simulink model "Test_model"  (R2021a)
settings: Solver=FixedStepDiscrete  StartTime=0.0  StopTime=10  RelTol=1e-3
values from neighbouring files (symbols this model uses):
  ADMM_vec = [ADMM_vec;ADMM_struct]    [Setup.m]
  constraints_struct = [constraints_struct;constraints]    [Setup.m]
undefined symbols (not defined in the file or in its folder): model, Objective
settings Model: SimulationMode=rapid-accelerator  Creator=worc4873  LastModifiedBy=worc4873
settings DebuggingCC: ReadBeforeWriteMsg=DisableAll  WriteAfterWriteMsg=DisableAll  WriteAfterReadMsg=DisableAll  MultiTaskDSMMsg=none
settings ModelReferenceCC: UpdateModelReferenceTargets=IfOutOfDate
settings SFSimCC: SFSimEcho=off

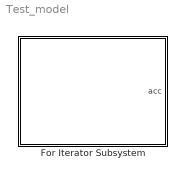
== system Test_model ==
  For Iterator Subsystem : Subsystem  TreatAsAtomicUnit=on

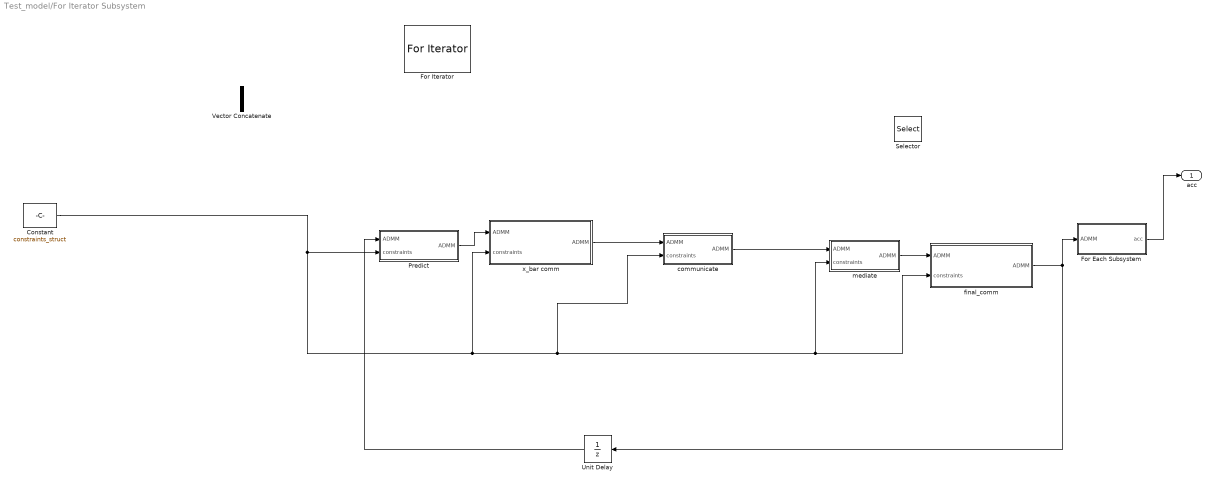
== system Test_model/For Iterator Subsystem ==
  Constant : Constant  Value=constraints_struct  OutDataTypeStr=Bus: constraints
  For Each Subsystem : Subsystem  TreatAsAtomicUnit=on
  For Iterator : ForIterator  IterationLimit=10
  Predict : Subsystem  TreatAsAtomicUnit=on
  Selector : Selector  InputPortWidth=3  IndexOptions=Index vector (dialog)  Indices=[1 3]  OutputSizes=1
  Unit Delay : UnitDelay  InitialCondition=ADMM_vec  SampleTime=-1  HasFrameUpgradeWarning=on
  Vector Concatenate : Concatenate
  communicate : Subsystem  TreatAsAtomicUnit=on
  final_comm : MATLAB Function  TreatAsAtomicUnit=on
  mediate : Subsystem  TreatAsAtomicUnit=on
  x_bar comm : MATLAB Function  TreatAsAtomicUnit=on
  acc : Outport
  wires:
  Constant/1 -> x_bar comm/2(constraints), final_comm/2(constraints), mediate/2(constraints), communicate/2(constraints), Predict/2(constraints)
  Predict/1(ADMM) -> x_bar comm/1("ADMM ")
  Unit Delay/1 -> Predict/1("ADMM ")
  x_bar comm/1(ADMM) -> communicate/1("ADMM ")
  communicate/1(ADMM) -> mediate/1("ADMM ")
  mediate/1(ADMM) -> final_comm/1("ADMM ")
  final_comm/1(ADMM) -> Unit Delay/1, For Each Subsystem/1(ADMM)
  For Each Subsystem/1(acc) -> acc/1

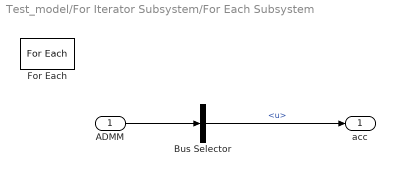
== system Test_model/For Iterator Subsystem/For Each Subsystem ==
  ADMM : Inport  Partition=on  PartitionDimension=1  PartitionWidth=1  PartitionOffset=0
  Bus Selector : BusSelector  OutputSignals=u
  For Each : ForEach  DisableCoverage=on
  acc : Outport  ConcatenationDimension=2
  wires:
  ADMM/1 -> Bus Selector/1
  Bus Selector/1 -> acc/1  "<u>"

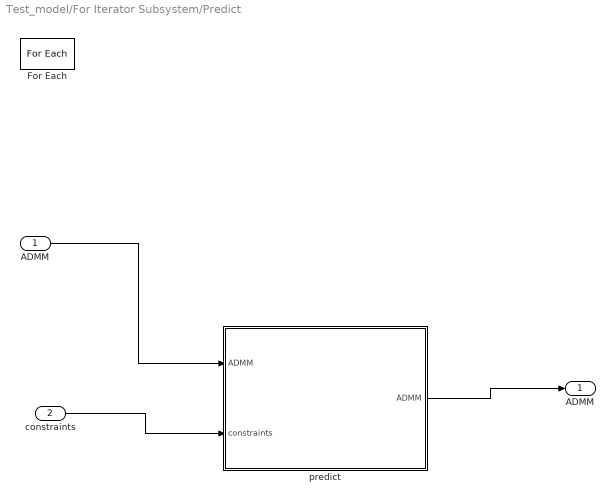
== system Test_model/For Iterator Subsystem/Predict ==
  "ADMM " : Inport  OutDataTypeStr=Bus: ADMM  Partition=on  PartitionDimension=1  PartitionWidth=1  PartitionOffset=0
  constraints : Inport  Port=2  OutDataTypeStr=Bus: constraints  Partition=on  PartitionDimension=1  PartitionWidth=1  PartitionOffset=0
  For Each : ForEach  DisableCoverage=on
  predict : MATLAB Function  TreatAsAtomicUnit=on
  ADMM : Outport  ConcatenationDimension=1
  wires:
  constraints/1 -> predict/2(constraints)
  "ADMM "/1 -> predict/1("ADMM ")
  predict/1(ADMM) -> ADMM/1

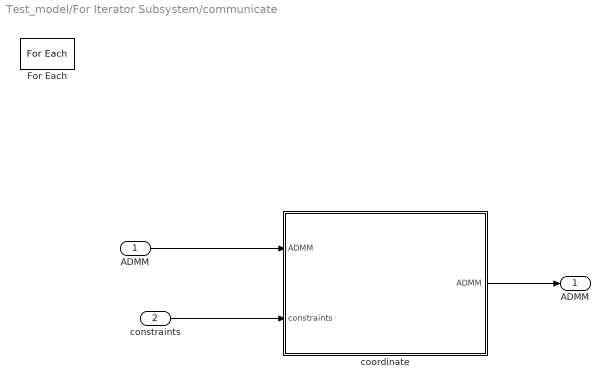
== system Test_model/For Iterator Subsystem/communicate ==
  "ADMM " : Inport  OutDataTypeStr=Bus: ADMM  Partition=on  PartitionDimension=1  PartitionWidth=1  PartitionOffset=0
  constraints : Inport  Port=2  OutDataTypeStr=Bus: constraints  Partition=on  PartitionDimension=1  PartitionWidth=1  PartitionOffset=0
  For Each : ForEach  DisableCoverage=on
  coordinate : MATLAB Function  TreatAsAtomicUnit=on
  ADMM : Outport  ConcatenationDimension=1
  wires:
  "ADMM "/1 -> coordinate/1("ADMM ")
  constraints/1 -> coordinate/2(constraints)
  coordinate/1(ADMM) -> ADMM/1

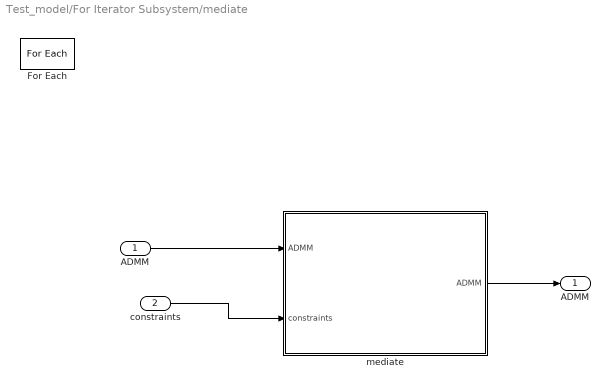
== system Test_model/For Iterator Subsystem/mediate ==
  "ADMM " : Inport  Partition=on  PartitionDimension=1  PartitionWidth=1  PartitionOffset=0
  constraints : Inport  Port=2  Partition=on  PartitionDimension=1  PartitionWidth=1  PartitionOffset=0
  For Each : ForEach  DisableCoverage=on
  mediate : MATLAB Function  TreatAsAtomicUnit=on
  ADMM : Outport  ConcatenationDimension=1
  wires:
  "ADMM "/1 -> mediate/1("ADMM ")
  constraints/1 -> mediate/2(constraints)
  mediate/1(ADMM) -> ADMM/1

== matlab function Test_model/For Iterator Subsystem/Predict/predict ==
  data: ADMM input Bus: ADMM; ADMM output; Objective parameter; model parameter; constraints input Bus: constraints
function ADMM = predict_step(ADMM,Objective, model, constraints)

Q = Objective.Q;
R = Objective.R;
N = Objective.N;

Nd = 3;
nx = size(Q,1);
nu = size(R,1);

A = model.A;
B = model.B;
umax = model.umax;
umin = model.umin;


N_j = constraints.N_j;
r = constraints.r;
x0 = constraints.x0;

rho = ADMM.rho;
lambda = ADMM.lambda;
lambda_from_j = ADMM.lambda_from_j;
w = ADMM.w;
w_from_j = ADMM.w_from_j;

min_input = repmat(ones(nu,1)*umin,N,1);
max_input = repmat(ones(nu,1)*umax,N,1);
% - linear dynamics

u_bound = [inf((N+1)*nx,1);max_input];
l_bound = [-inf((N+1)*nx,1);min_input];


posM = blkdiag(eye(Nd),zeros(nx-Nd)); % Matrix to take only position from the state vector x (zeros rest)
d = [eye(Nd),zeros(Nd,nx-Nd)]; % Matrix to take only position from the state vector x (only returns pos)
posMN = kron(eye(N+1),d); %returns pos across time steps

Ax = kron(speye(N+1), -speye(nx)) + kron(sparse(diag(ones(N, 1), -1)), A);
Bu = kron([sparse(1, N); speye(N)], B);
Aeq = [Ax, Bu];
b_eq = [-x0'; zeros(N*nx, 1)];
P_new = blkdiag( kron(eye(N), Q+ (size(N_j,2)+1)*rho/2*posM ), Q+(size(N_j,2)+1)*rho/2*posM, kron(eye(N), R) );

q = prediction_linear(lambda,lambda_from_j,w,w_from_j,rho,r',Q,N,nu,posMN);

qp_opts = optimoptions('quadprog','Display','off','Algorithm','active-set');
init = [ADMM.x;ADMM.u];
res = quadprog(P_new,q,[],[], full(Aeq),b_eq,l_bound,u_bound,init,qp_opts);
ADMM.x = res(1:nx*(N+1));
ADMM.u = res((N+1)*nx+1:end);

end

== matlab function Test_model/For Iterator Subsystem/x_bar comm ==
  data: ADMM input Bus: ADMM; ADMM output; constraints input Bus: constraints
function ADMM = comm_xbar(ADMM,constraints)

for i =1:size(ADMM,1)
    ADMM(i).x_bar(:,1) = ADMM(i).x;
    for j = 1:size(constraints(i).N_j,2)
        ADMM(i).x_bar(:,j+1) = ADMM(constraints(i).N_j(j)).x;
    end
end

== matlab function Test_model/For Iterator Subsystem/final_comm ==
  data: ADMM input Bus: ADMM; ADMM output; constraints input Bus: constraints
function ADMM = final_comm(ADMM,constraints)

    for i = 1:size(ADMM,1)
        for j = 1:size(constraints(i).N_j,2)
            curr_comm = constraints(i).N_j(j);
            ADMM(i).lambda_from_j(:,j) = ADMM(curr_comm).lambda_to_j(:,(constraints(curr_comm).N_j==i));
            ADMM(i).w_from_j(:,j) = ADMM(curr_comm).w_to_j(:,(constraints(curr_comm).N_j==i));
        end
        
    end

== matlab function Test_model/For Iterator Subsystem/communicate/coordinate ==
  data: ADMM input Bus: ADMM; ADMM output; Objective parameter; constraints input Bus: constraints
function ADMM = coordinate_step(ADMM,Objective, constraints)

Nd = 3;
nx = size(Objective.Q,1);
nu = size(Objective.R,1);

N = Objective.N;

d = [eye(Nd),zeros(Nd,nx-Nd)]; % Matrix to take only position from the state vector x (only returns pos)
posMN = kron(eye(N+1),d); %returns pos across time steps


rhoM = kron(speye((N+1)),ADMM.rho/2*eye(nu)); % matrix for the quadratic objective formualation
Pc = kron(eye(1+size(constraints.N_j,2)),rhoM);

H = kron(eye(N+1),repmat(d, size(constraints.N_j,2), 1));
Hw = kron(eye(N+1),repmat(eye(nu), size(constraints.N_j,2), 1));
for j = 1:size(constraints.N_j,2)
    v = zeros(size(constraints.N_j,2),1);
    v(j) = 1;
    H_M = kron(eye(N+1),kron(v, -1*d));
    H_Mw = kron(eye(N+1),kron(v, -1*eye(nu)));
    
    H =  [H, H_M];
    Hw = [Hw,H_Mw];
end
qc = coordination_linear(ADMM.lambda,ADMM.lambda_to_j,ADMM.rho,ADMM.x_bar,posMN);

% Update matrices

qp_opts = optimoptions('quadprog','Display','off','Algorithm','active-set');
init = ADMM.w;
for j = 1:size(constraints.N_j,2)
   init = [init;ADMM.w_to_j(:,j)]; 
end
[A_ineq,l_ineq] = communicate(ADMM.x_bar,Objective.N,constraints.N_j,H,Hw,constraints.delta,nu);
resc = quadprog(full(Pc),qc,-A_ineq,-l_ineq,[],[],[],[],init,qp_opts);


ADMM.w = resc(1:Nd*(N+1),1);
for j = 1:size(constraints.N_j,2)
    ADMM.w_to_j(:,j) = resc(j*Nd*(N+1)+1:(j+1)*Nd*(N+1),1);
end

end

== matlab function Test_model/For Iterator Subsystem/mediate/mediate ==
  data: ADMM input Bus: ADMM; ADMM output; N parameter; constraints input Bus: constraints
function ADMM = mediate_step(ADMM,N, constraints)

Nd = 3;
nx = size(ADMM.x,1)/(N+1);

d = [eye(Nd),zeros(Nd,nx-Nd)]; % Matrix to take only position from the state vector x (only returns pos)
posMN = kron(eye(N+1),d); %returns pos across time steps


ADMM.lambda = ADMM.lambda + ADMM.rho * (posMN * ADMM.x-ADMM.w);
for j = 1:size(constraints.N_j,2)
    ADMM.lambda_to_j(:,j) = ADMM.lambda_to_j(:,j) + ADMM.rho * (posMN*ADMM.x_bar(:,j+1) - ADMM.w_to_j(:,j));
end

end
